simulink model "motorai"  (R2018b)
settings: Solver=FixedStepAuto  StartTime=0.0  StopTime=inf  FixedStep=SAMPLE_TIME  RelTol=1e-3
PreLoadFcn:
  | UserSettings
InitFcn:
  | ESTIMATION_SAMPLES = 50;
values from neighbouring files (symbols this model uses):
  ADC_bits = 12    [LQR_control_design.m]    (also in UserSettings.m)
  ADC_Vref = 3.3    [LQR_control_design.m]    (also in UserSettings.m)
  current_gain = 0.5    [LQR_control_design.m]    (also in UserSettings.m)
  current_offset = 1    [LQR_control_design.m]    (also in UserSettings.m)
  DATA_SAMPLING_FREQUENCY = 500    [UserSettings.m]
  K = -K    (= -0.383)    [LQG_control_design.m]    (also in LQR_control_design.m = -(1/R).*B'*Sinf; myLQR.m = -(1/R).*B'*Sinf; myREF.m = [Kw Ki])
  motorParameters = Parameters()    [UserSettings.m]
  omega_gain = 0.5    [LQR_control_design.m]    (also in UserSettings.m)
  omega_offset = 1    [LQR_control_design.m]    (also in UserSettings.m)
  PPR = 1000    [LQR_control_design.m]    (also in UserSettings.m)
  Q = 1/2*inv([(omega_max)^2 0 0; 0 (i_max)^2 0; 0 0 (int_max)^2])    [LQG_control_design.m]    (also in LQR_control_design.m = 1/2*inv([(omega_max)^2 0 ; 0 (i_max)^2]); myLQR.m = 1/2*inv([(omega_max)^2 0; 0 (i_max)^2]))
  R = inv([(v_max)^2])    [LQG_control_design.m]    (also in LQR_control_design.m; myLQR.m)
  SAMPLE_TIME = 5e-5    (= 5e-05)    [UserSettings.m]
  V_ACT = 12    [UserSettings.m]
  Vact = 12    [LQR_control_design.m]
undefined symbols (not defined in the file or in its folder): DiscIntNeverNeededParam
libraries: neural x275, mbedblockslib x7, fl_lib x5, nesl_utility x5, dspswit3 x3, elec_lib x3, powerlib_meascontrol x3, dspbuff3 x2, discretizing x1
(part 4 of 14)

== system motorai/PARAMETERS EXTIMATION HIL/Function Fitting Neural Network/Layer 2/Delays 1 ==
  "p{2}" : Inport  PortDimensions=22
      mask Display: e = 0.06;c1 = [120 230 180]/255;c2 = ([120 230 180]+0)/(256+128);c3 = ([120 230 180]+128)/(256+128);patch([0 1 1 0],[0 0 1 1],c1);patch([0 1 1 1-e 1-e 0+e],[0 0 1 1-e 0+e 0+e],c2);patch([0 0 1 1-e 0+e 0+e],[0 1 1 1-e 1-e 0+e],c3);plot([0 1 1 0 0],[0 0 1 1 0]);
  mux : Mux  Inputs=1
      mask Display: e = 0.06;c1 = [120 150 230]/255;c2 = ([120 150 230]+0)/383;c3 = ([120 150 230]+128)/383;patch([0 1 1 0],[0 0 1 1],c1);patch([0 1 1 1-e 1-e 0+e],[0 0 1 1-e 0+e 0+e],c2);patch([0 0 1 1-e 0+e 0+e],[0 1 1 1-e 1-e 0+e],c3);plot([0 1 1 0 0],[0 0 1 1 0]);disp('Mux')
  "pd{2,1}" : Outport
      mask Display: e = 0.06;c1 = [120 230 180]/255;c2 = ([120 230 180]+0)/(256+128);c3 = ([120 230 180]+128)/(256+128);patch([0 1 1 0],[0 0 1 1],c1);patch([0 1 1 1-e 1-e 0+e],[0 0 1 1-e 0+e 0+e],c2);patch([0 0 1 1-e 0+e 0+e],[0 1 1 1-e 1-e 0+e],c3);plot([0 1 1 0 0],[0 0 1 1 0]);
  wires:
  mux/1 -> "pd{2,1}"/1
  "p{2}"/1 -> mux/1

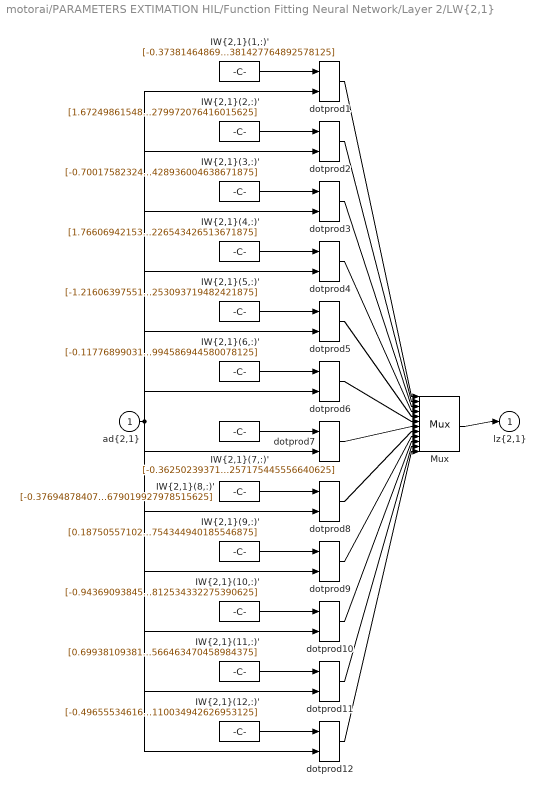
== system motorai/PARAMETERS EXTIMATION HIL/Function Fitting Neural Network/Layer 2/LW{2,1} ==
  "ad{2,1}" : Inport  PortDimensions=22
      mask Display: e = 0.06;c1 = [120 230 180]/255;c2 = ([120 230 180]+0)/(256+128);c3 = ([120 230 180]+128)/(256+128);patch([0 1 1 0],[0 0 1 1],c1);patch([0 1 1 1-e 1-e 0+e],[0 0 1 1-e 0+e 0+e],c2);patch([0 0 1 1-e 0+e 0+e],[0 1 1 1-e 1-e 0+e],c3);plot([0 1 1 0 0],[0 0 1 1 0]);
  "IW{2,1}(1,:)'" : Constant  Value=[-0.373814648698248042091307752343709580600261688232421875;2.388185086648772159634290801477618515491485595703125;0.306022187467772710522950774247874505817890167236328125;-0.74612148152227353303800327921635471284389495849609375;-0.36510707287944976773275129744433797895908355712890625;0.3483392363810693392878192753414623439311981201171875;1.0579275570388186888948212072136811912059783935546875;0.293660952316886436630483103726874105632305145263671875;2.12653508516325917554468105663545429706573486328125;0.66856009697980989248122796198003925383090972900390625;-0.51653241823746720573495849748724140226840972900390625;-0.62461964538400105428905817461782135069370269775390625;0.73347032324756289423106636604643426835536956787109375;0.60107951005838733404829099526978097856044769287109375;0.41661190433255190779249232946312986314296722412109375;-0.495062523768045215089017574427998624742031097412109375;-0.97392836170859575783964601214393042027950286865234375;-0.15328348744030317885034264691057614982128143310546875;0.955526268447108417802837720955722033977508544921875;0.30437862753427535889017008230439387261867523193359375;3.0866869361023301365776205784641206264495849609375;-0.4803399659008598110432330940966494381427764892578125]
      mask Display: e = 0.06;c1 = [120 150 230]/255;c2 = ([120 150 230]+0)/383;c3 = ([120 150 230]+128)/383;patch([0 1 1 0],[0 0 1 1],c1);patch([0 1 1 1-e 1-e 0+e],[0 0 1 1-e 0+e 0+e],c2);patch([0 0 1 1-e 0+e 0+e],[0 1 1 1-e 1-e 0+e],c3);plot([0 1 1 0 0],[0 0 1 1 0]);disp('weights');
  "IW{2,1}(10,:)'" : Constant  Value=[-0.94369093845881446558365723831229843199253082275390625;1.322843320356273721927209408022463321685791015625;0.2013525000172964596334423958978732116520404815673828125;-0.429323077932844909820886414308915846049785614013671875;0.1744635303798653114260019947323598898947238922119140625;-0.041808522872746757548245710722767398692667484283447265625;-0.210001538457013026128805677217314951121807098388671875;0.157787948169038128032326540051144547760486602783203125;-0.59934844013664434481114540176349692046642303466796875;0.0142991425154821438781027609365992248058319091796875;1.8154415812965656318311857830849476158618927001953125;-0.2181115352241077831596527403235086239874362945556640625;-0.7770603432838161239715191186405718326568603515625;0.4534919681510520828027210882282815873622894287109375;-0.237948861224295205030188071759766899049282073974609375;-1.6341662334094799735595415768329985439777374267578125;0.59471843043654015747989660667371936142444610595703125;0.727832247307649282674901769496500492095947265625;0.1267307587950488312333874318937887437641620635986328125;1.2978618628956042346800359155167825520038604736328125;-2.018836157679956944122068307478912174701690673828125;0.304437176117283991860773539883666671812534332275390625]
      mask Display: e = 0.06;c1 = [120 150 230]/255;c2 = ([120 150 230]+0)/383;c3 = ([120 150 230]+128)/383;patch([0 1 1 0],[0 0 1 1],c1);patch([0 1 1 1-e 1-e 0+e],[0 0 1 1-e 0+e 0+e],c2);patch([0 0 1 1-e 0+e 0+e],[0 1 1 1-e 1-e 0+e],c3);plot([0 1 1 0 0],[0 0 1 1 0]);disp('weights');
  "IW{2,1}(11,:)'" : Constant  Value=[0.6993810938157587475672016807948239147663116455078125;-19.28028374521506549399418872781097888946533203125;2.309346273318040321242960999370552599430084228515625;1.0652462012675394387173355426057241857051849365234375;-2.145760240313183242477634848910383880138397216796875;3.155749157418584527334814993082545697689056396484375;1.1460430072098544140857256934395991265773773193359375;-0.03602755514596193975318527691342751495540142059326171875;7.37193274662607489489118961500935256481170654296875;2.910634893704704406758310142322443425655364990234375;-2.502679544920492826776126094046048820018768310546875;5.475021714965532027008521254174411296844482421875;-2.190915873696507976120528837782330811023712158203125;0.40460150291473684358578566389041952788829803466796875;7.06424053190595113704830509959720075130462646484375;-2.498408304964217396815229221829213201999664306640625;-1.66854689838172287608131227898411452770233154296875;4.956010968949474460032433853484690189361572265625;-0.9894118095536430512737524622934870421886444091796875;3.398294550650808876213204712257720530033111572265625;-6.42259294605289188240249131922610104084014892578125;-1.01288980257130756257311077206395566463470458984375]
      mask Display: e = 0.06;c1 = [120 150 230]/255;c2 = ([120 150 230]+0)/383;c3 = ([120 150 230]+128)/383;patch([0 1 1 0],[0 0 1 1],c1);patch([0 1 1 1-e 1-e 0+e],[0 0 1 1-e 0+e 0+e],c2);patch([0 0 1 1-e 0+e 0+e],[0 1 1 1-e 1-e 0+e],c3);plot([0 1 1 0 0],[0 0 1 1 0]);disp('weights');
  "IW{2,1}(12,:)'" : Constant  Value=[-0.496555346166215938463750489972881041467189788818359375;0.00791055524906490899195166122126465779729187488555908203125;-0.11710097566626261056388358383628656156361103057861328125;-0.0165177005587808893583012803674137103371322154998779296875;-0.6454360744191973697780895236064679920673370361328125;-0.6732070109779215716372391398181207478046417236328125;0.09373162307416758876055240534697077237069606781005859375;-0.039114682492637047050987320062631624750792980194091796875;-0.1551113925473206200944531474306131713092327117919921875;-0.05012488071425476310327695728119579143822193145751953125;0.2156283243173235941725351949571631848812103271484375;-0.8022298048740685860735766254947520792484283447265625;-0.9063317432573414489382912506698630750179290771484375;-0.00032101082763222560205462752236371670733205974102020263671875;0.2671447035854070950477989754290319979190826416015625;0.69691015959264646095761008837143890559673309326171875;-0.1784561380273828878895159277817583642899990081787109375;-0.05347038743792344173133557205801480449736118316650390625;-0.11345954903014165982000349686131812632083892822265625;0.01728629936978050285478758496537921018898487091064453125;-0.85915203372011827998022681640577502548694610595703125;-1.5394571537418759721305150378611870110034942626953125]
      mask Display: e = 0.06;c1 = [120 150 230]/255;c2 = ([120 150 230]+0)/383;c3 = ([120 150 230]+128)/383;patch([0 1 1 0],[0 0 1 1],c1);patch([0 1 1 1-e 1-e 0+e],[0 0 1 1-e 0+e 0+e],c2);patch([0 0 1 1-e 0+e 0+e],[0 1 1 1-e 1-e 0+e],c3);plot([0 1 1 0 0],[0 0 1 1 0]);disp('weights');
  "IW{2,1}(2,:)'" : Constant  Value=[1.67249861548387013243655019323341548442840576171875;-0.0501570542810379771392348402514471672475337982177734375;5.45446144012502553977128627593629062175750732421875;0.3067453305420440035078399887424893677234649658203125;0.93388522037497179173470840396475978195667266845703125;0.43936786222361068343644774358836002647876739501953125;-0.72633915551496486262550433821161277592182159423828125;3.452667124378164142939340308657847344875335693359375;-1.1865375265624635847672152522136457264423370361328125;5.83346097285197284776359083480201661586761474609375;-0.7944995956295841654792866393108852207660675048828125;-1.39409214113267676538043815526179969310760498046875;-1.0713655944878925918573031594860367476940155029296875;-1.00512386920140972534909451496787369251251220703125;-1.5609895974406218233099252756801433861255645751953125;-2.43147394289584628523925857734866440296173095703125;-2.897976439331302334068141135503537952899932861328125;-2.880108124462474439297920980607159435749053955078125;11.235313175654884076948292204178869724273681640625;-1.5185828429420393792526056131464429199695587158203125;-3.28633815506999216182748568826355040073394775390625;12.7821791830810784773575505823828279972076416015625]
      mask Display: e = 0.06;c1 = [120 150 230]/255;c2 = ([120 150 230]+0)/383;c3 = ([120 150 230]+128)/383;patch([0 1 1 0],[0 0 1 1],c1);patch([0 1 1 1-e 1-e 0+e],[0 0 1 1-e 0+e 0+e],c2);patch([0 0 1 1-e 0+e 0+e],[0 1 1 1-e 1-e 0+e],c3);plot([0 1 1 0 0],[0 0 1 1 0]);disp('weights');
  "IW{2,1}(3,:)'" : Constant  Value=[-0.70017582324454863407225957416812889277935028076171875;1.67067467675322323117370615364052355289459228515625;0.1254376935351457500456007210232201032340526580810546875;-0.496595212722104661917654766511986963450908660888671875;0.094918003618071844496029143556370399892330169677734375;0.264165279391440355194475841926760040223598480224609375;-0.139597218341219797554941806083661504089832305908203125;0.117080505236092979881590281365788541734218597412109375;-0.55579337936531036934439953256514854729175567626953125;0.01236978846688709283985208031708680209703743457794189453125;1.4945214065591017060796730220317840576171875;-0.0880529371837325547378583223689929582178592681884765625;-0.7157812903296789652785037105786614120006561279296875;0.3810758435795695842074337633675895631313323974609375;-0.26285342121100196965954864936065860092639923095703125;-0.812099360289087801589857917861081659793853759765625;0.53431861847600747861264380844659171998500823974609375;0.7215442121609945136384567376808263361454010009765625;0.04721860197450167273558463421068154275417327880859375;1.1988879951099453702312302993959747254848480224609375;-3.33608458289905396298991036019288003444671630859375;-0.7836158906533199353106056150863878428936004638671875]
      mask Display: e = 0.06;c1 = [120 150 230]/255;c2 = ([120 150 230]+0)/383;c3 = ([120 150 230]+128)/383;patch([0 1 1 0],[0 0 1 1],c1);patch([0 1 1 1-e 1-e 0+e],[0 0 1 1-e 0+e 0+e],c2);patch([0 0 1 1-e 0+e 0+e],[0 1 1 1-e 1-e 0+e],c3);plot([0 1 1 0 0],[0 0 1 1 0]);disp('weights');
  "IW{2,1}(4,:)'" : Constant  Value=[1.766069421533778882604792670463211834430694580078125;1.042967917183602377662055005203001201152801513671875;-0.141883868596699047603948429241427220404148101806640625;-0.58806106441775085613699047826230525970458984375;0.311817283999389294191217913976288400590419769287109375;2.3102000569721088396590857882983982563018798828125;4.15528975409117862227503792382776737213134765625;6.21171473959054143421099070110358297824859619140625;0.1196618271109388953465924032570910640060901641845703125;0.11815122529796819039749067314915009774267673492431640625;0.9828675247137164117106067351414822041988372802734375;-1.2034037682147538106391948531381785869598388671875;-0.152664932005876163856328275869600474834442138671875;-4.595335314922895264544422389008104801177978515625;-0.6266982814945289970154362890752963721752166748046875;-1.1989185909846666877598408973426558077335357666015625;-3.6425990245676214129844083799980580806732177734375;0.123378486656041952418405571734183467924594879150390625;0.173975621097830324135458113232743926346302032470703125;-1.266562415572969779731238304520957171916961669921875;3.385659680429013551616890254081226885318756103515625;-2.130314063352613640489607860217802226543426513671875]
      mask Display: e = 0.06;c1 = [120 150 230]/255;c2 = ([120 150 230]+0)/383;c3 = ([120 150 230]+128)/383;patch([0 1 1 0],[0 0 1 1],c1);patch([0 1 1 1-e 1-e 0+e],[0 0 1 1-e 0+e 0+e],c2);patch([0 0 1 1-e 0+e 0+e],[0 1 1 1-e 1-e 0+e],c3);plot([0 1 1 0 0],[0 0 1 1 0]);disp('weights');
  "IW{2,1}(5,:)'" : Constant  Value=[-1.2160639755125342009733913073432631790637969970703125;-3.038322807923126589457751833833754062652587890625;2.95356675575607408035239132004790008068084716796875;-0.34964856620207240833764217313728295266628265380859375;-3.8401663498015086162240550038404762744903564453125;-1.434312482104028507734483355307020246982574462890625;0.498000988776814867975417655543424189090728759765625;-0.475940354291554623689108893813681788742542266845703125;0.481776521841532356926762759030680172145366668701171875;-0.0143285253932178245628303869807496084831655025482177734375;-1.62541639988879449418845979380421340465545654296875;-1.33097413271977504933829550282098352909088134765625;1.1551325139709671674381752382032573223114013671875;0.322054940956319313283273686465690843760967254638671875;0.83090978260683778788830977646284736692905426025390625;-0.9638347486264853269943841951317153871059417724609375;-0.17447941373044584256746247774572111666202545166015625;-1.6259520001337108840999690073658712208271026611328125;-0.0201962158267790063692626034708155202679336071014404296875;-2.034125459290754722729843706474639475345611572265625;7.29613836782051183860176024609245359897613525390625;-1.7639138340141122807125384497339837253093719482421875]
      mask Display: e = 0.06;c1 = [120 150 230]/255;c2 = ([120 150 230]+0)/383;c3 = ([120 150 230]+128)/383;patch([0 1 1 0],[0 0 1 1],c1);patch([0 1 1 1-e 1-e 0+e],[0 0 1 1-e 0+e 0+e],c2);patch([0 0 1 1-e 0+e 0+e],[0 1 1 1-e 1-e 0+e],c3);plot([0 1 1 0 0],[0 0 1 1 0]);disp('weights');
  "IW{2,1}(6,:)'" : Constant  Value=[-0.11776899031336483802956394129068939946591854095458984375;1.0816067725283800005087186946184374392032623291015625;-1.3725069564608916028447538337786681950092315673828125;-0.93885172581776288325272616930305957794189453125;-0.334927153732878346570345229338272474706172943115234375;3.127055083824247905255333535023964941501617431640625;3.737129929311676423964172499836422502994537353515625;6.57794136604749812846648637787438929080963134765625;0.18819194287160512235601572683663107454776763916015625;0.0062255822559748770494980618650515680201351642608642578125;1.39585907348498050595253516803495585918426513671875;-0.85890284540357908493746208478114567697048187255859375;-2.17788422026401207176604657433927059173583984375;-4.8394935373831469149763506720773875713348388671875;-0.63340718588441635716890232288278639316558837890625;-5.893111992691302702951361425220966339111328125;-2.575737579748121230949209348182193934917449951171875;0.1688019695557121391260579912341199815273284912109375;0.0131168749563965840454482503218969213776290416717529296875;-2.832832085014937550937474952661432325839996337890625;8.6321982981284204328176201670430600643157958984375;-3.655848587658077963880032257293350994586944580078125]
      mask Display: e = 0.06;c1 = [120 150 230]/255;c2 = ([120 150 230]+0)/383;c3 = ([120 150 230]+128)/383;patch([0 1 1 0],[0 0 1 1],c1);patch([0 1 1 1-e 1-e 0+e],[0 0 1 1-e 0+e 0+e],c2);patch([0 0 1 1-e 0+e 0+e],[0 1 1 1-e 1-e 0+e],c3);plot([0 1 1 0 0],[0 0 1 1 0]);disp('weights');
  "IW{2,1}(7,:)'" : Constant  Value=[-0.3625023937196261147875020469655282795429229736328125;2.741236662902159171295579653815366327762603759765625;-2.121606761392355711137724938453175127506256103515625;-0.4523900379543508432078624537098221480846405029296875;-1.433230340797343682623932181741110980510711669921875;1.878588877026521775093215183005668222904205322265625;-0.560815005670500799084265963756479322910308837890625;1.493913929936840911949502697098068892955780029296875;-3.170568963376355409167217658250592648983001708984375;4.33352532635525466986337050911970436573028564453125;-1.0881674978698507860741528929793275892734527587890625;0.5463363153126630233913374468102119863033294677734375;1.070531714404931111772611984633840620517730712890625;-0.6797290363552226377663600942469201982021331787109375;-3.36627763772676313891452082316391170024871826171875;0.131098898813111708339107508436427451670169830322265625;-1.17719923016618022160173495649360120296478271484375;3.258685294179720859375493091647513210773468017578125;5.725185804640826603417735896073281764984130859375;-1.5388387016591653644326243011164478957653045654296875;8.124922737557515262096785590983927249908447265625;3.238888438369118549786662697442807257175445556640625]
      mask Display: e = 0.06;c1 = [120 150 230]/255;c2 = ([120 150 230]+0)/383;c3 = ([120 150 230]+128)/383;patch([0 1 1 0],[0 0 1 1],c1);patch([0 1 1 1-e 1-e 0+e],[0 0 1 1-e 0+e 0+e],c2);patch([0 0 1 1-e 0+e 0+e],[0 1 1 1-e 1-e 0+e],c3);plot([0 1 1 0 0],[0 0 1 1 0]);disp('weights');
  "IW{2,1}(8,:)'" : Constant  Value=[-0.376948784072008435952483296205173246562480926513671875;-2.744608844334838426703981895116157829761505126953125;-0.354979565149837028581458753251354210078716278076171875;0.5446501025508629911797697786823846399784088134765625;0.52623456523853373578702985469135455787181854248046875;-0.4870280253021739280683277684147469699382781982421875;-0.94904641297388481202546017811982892453670501708984375;-0.27048626906591000107482614112086594104766845703125;-0.1371915607268853476430336968405754305422306060791015625;-0.5775952934599619670308356944588012993335723876953125;0.460047851461393264571597683243453502655029296875;-0.458507355789205206519909552298486232757568359375;-0.81339419741809682040667439650860615074634552001953125;-0.5181965606424674408714281526044942438602447509765625;1.446283776482689464870645679184235632419586181640625;-0.2037852020641963690650300122797489166259765625;1.03066658521672405157687535393051803112030029296875;-4.4452367691895613432961908983998000621795654296875;-0.9924712041404737394856283572153188288211822509765625;-0.19396147486783277269495329164783470332622528076171875;-2.33074689468901841138404051889665424823760986328125;2.7750555478774376894079978228546679019927978515625]
      mask Display: e = 0.06;c1 = [120 150 230]/255;c2 = ([120 150 230]+0)/383;c3 = ([120 150 230]+128)/383;patch([0 1 1 0],[0 0 1 1],c1);patch([0 1 1 1-e 1-e 0+e],[0 0 1 1-e 0+e 0+e],c2);patch([0 0 1 1-e 0+e 0+e],[0 1 1 1-e 1-e 0+e],c3);plot([0 1 1 0 0],[0 0 1 1 0]);disp('weights');
  "IW{2,1}(9,:)'" : Constant  Value=[0.1875055710261027408503053948152228258550167083740234375;0.90489674608045189696525767431012354791164398193359375;-0.12973322723757008123612877170671708881855010986328125;0.4040789428277340444850551648414693772792816162109375;0.7588494540475922978117750972160138189792633056640625;0.22043493779026090972905649323365651071071624755859375;0.091262840672618195103638072396279312670230865478515625;-0.10358510239831585086900389569564140401780605316162109375;0.48469536828752846080448080101632513105869293212890625;-0.1042448443682677805544045668284525163471698760986328125;-2.28001013511277950129851888050325214862823486328125;-0.401620072308292275220509282007697038352489471435546875;0.5889009231164286095605575610534287989139556884765625;-0.428874131242132694552537941490299999713897705078125;0.426953858134898556198066899014520458877086639404296875;3.73162300623667153587348366272635757923126220703125;-0.56022450979731319709031822640099562704563140869140625;-0.7703389604056589679004218851332552731037139892578125;-0.152647405145999337516826699356897734105587005615234375;-1.03590236727699736007934916415251791477203369140625;-0.54521841184197306073855315844411961734294891357421875;-4.37328944251520379538078486802987754344940185546875]
      mask Display: e = 0.06;c1 = [120 150 230]/255;c2 = ([120 150 230]+0)/383;c3 = ([120 150 230]+128)/383;patch([0 1 1 0],[0 0 1 1],c1);patch([0 1 1 1-e 1-e 0+e],[0 0 1 1-e 0+e 0+e],c2);patch([0 0 1 1-e 0+e 0+e],[0 1 1 1-e 1-e 0+e],c3);plot([0 1 1 0 0],[0 0 1 1 0]);disp('weights');
  Mux : Mux  Inputs=12
      mask Display: e = 0.06;c1 = [120 150 230]/255;c2 = ([120 150 230]+0)/383;c3 = ([120 150 230]+128)/383;patch([0 1 1 0],[0 0 1 1],c1);patch([0 1 1 1-e 1-e 0+e],[0 0 1 1-e 0+e 0+e],c2);patch([0 0 1 1-e 0+e 0+e],[0 1 1 1-e 1-e 0+e],c3);plot([0 1 1 0 0],[0 0 1 1 0]);disp('Mux');
  dotprod{1..12} (12 alike) : neural/Weight Functions/dotprod
      settings: SourceProductName=Deep Learning Toolbox
  "lz{2,1}" : Outport
      mask Display: e = 0.06;c1 = [120 230 180]/255;c2 = ([120 230 180]+0)/(256+128);c3 = ([120 230 180]+128)/(256+128);patch([0 1 1 0],[0 0 1 1],c1);patch([0 1 1 1-e 1-e 0+e],[0 0 1 1-e 0+e 0+e],c2);patch([0 0 1 1-e 0+e 0+e],[0 1 1 1-e 1-e 0+e],c3);plot([0 1 1 0 0],[0 0 1 1 0]);
  wires:
  Mux/1 -> "lz{2,1}"/1
  dotprod12/1 -> Mux/12
  "IW{2,1}(12,:)'"/1 -> dotprod12/1
  dotprod11/1 -> Mux/11
  "IW{2,1}(11,:)'"/1 -> dotprod11/1
  dotprod10/1 -> Mux/10
  "IW{2,1}(10,:)'"/1 -> dotprod10/1
  dotprod9/1 -> Mux/9
  "IW{2,1}(9,:)'"/1 -> dotprod9/1
  dotprod8/1 -> Mux/8
  "IW{2,1}(8,:)'"/1 -> dotprod8/1
  dotprod7/1 -> Mux/7
  "IW{2,1}(7,:)'"/1 -> dotprod7/1
  dotprod6/1 -> Mux/6
  "IW{2,1}(6,:)'"/1 -> dotprod6/1
  dotprod5/1 -> Mux/5
  "IW{2,1}(5,:)'"/1 -> dotprod5/1
  dotprod4/1 -> Mux/4
  "IW{2,1}(4,:)'"/1 -> dotprod4/1
  dotprod3/1 -> Mux/3
  "IW{2,1}(3,:)'"/1 -> dotprod3/1
  dotprod2/1 -> Mux/2
  "IW{2,1}(2,:)'"/1 -> dotprod2/1
  dotprod1/1 -> Mux/1
  "ad{2,1}"/1 -> dotprod12/2, dotprod11/2, dotprod10/2, dotprod9/2, dotprod8/2, dotprod7/2, dotprod6/2, dotprod5/2, dotprod4/2, dotprod3/2, dotprod2/2, dotprod1/2
  "IW{2,1}(1,:)'"/1 -> dotprod1/1

== system motorai/PARAMETERS EXTIMATION HIL/Function Fitting Neural Network/Layer 3/Delays 1 ==
  "p{3}" : Inport  PortDimensions=12
      mask Display: e = 0.06;c1 = [120 230 180]/255;c2 = ([120 230 180]+0)/(256+128);c3 = ([120 230 180]+128)/(256+128);patch([0 1 1 0],[0 0 1 1],c1);patch([0 1 1 1-e 1-e 0+e],[0 0 1 1-e 0+e 0+e],c2);patch([0 0 1 1-e 0+e 0+e],[0 1 1 1-e 1-e 0+e],c3);plot([0 1 1 0 0],[0 0 1 1 0]);
  mux : Mux  Inputs=1
      mask Display: e = 0.06;c1 = [120 150 230]/255;c2 = ([120 150 230]+0)/383;c3 = ([120 150 230]+128)/383;patch([0 1 1 0],[0 0 1 1],c1);patch([0 1 1 1-e 1-e 0+e],[0 0 1 1-e 0+e 0+e],c2);patch([0 0 1 1-e 0+e 0+e],[0 1 1 1-e 1-e 0+e],c3);plot([0 1 1 0 0],[0 0 1 1 0]);disp('Mux')
  "pd{3,2}" : Outport
      mask Display: e = 0.06;c1 = [120 230 180]/255;c2 = ([120 230 180]+0)/(256+128);c3 = ([120 230 180]+128)/(256+128);patch([0 1 1 0],[0 0 1 1],c1);patch([0 1 1 1-e 1-e 0+e],[0 0 1 1-e 0+e 0+e],c2);patch([0 0 1 1-e 0+e 0+e],[0 1 1 1-e 1-e 0+e],c3);plot([0 1 1 0 0],[0 0 1 1 0]);
  wires:
  mux/1 -> "pd{3,2}"/1
  "p{3}"/1 -> mux/1

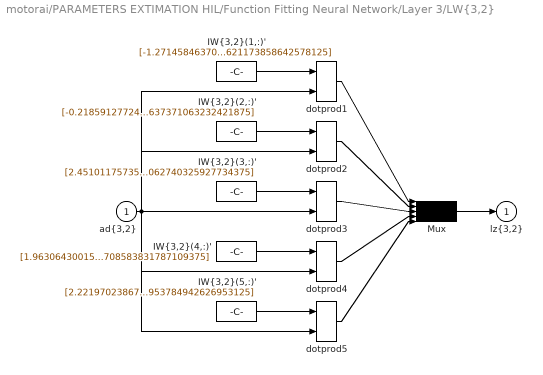
== system motorai/PARAMETERS EXTIMATION HIL/Function Fitting Neural Network/Layer 3/LW{3,2} ==
  "ad{3,2}" : Inport  PortDimensions=12
      mask Display: e = 0.06;c1 = [120 230 180]/255;c2 = ([120 230 180]+0)/(256+128);c3 = ([120 230 180]+128)/(256+128);patch([0 1 1 0],[0 0 1 1],c1);patch([0 1 1 1-e 1-e 0+e],[0 0 1 1-e 0+e 0+e],c2);patch([0 0 1 1-e 0+e 0+e],[0 1 1 1-e 1-e 0+e],c3);plot([0 1 1 0 0],[0 0 1 1 0]);
  "IW{3,2}(1,:)'" : Constant  Value=[-1.271458463700293695097798263304866850376129150390625;-0.8974504950343582532212849400821141898632049560546875;-1.7160155942908417170400525719742290675640106201171875;3.778124449975665211098885265528224408626556396484375;1.0463511136165484227689148610807023942470550537109375;-4.198289194390252276889441418461501598358154296875;2.185971342736543032714280343498103320598602294921875;-1.562305785175263306285842190845869481563568115234375;2.086082505458115132768170951749198138713836669921875;3.74283631710132880243691033683717250823974609375;0.50886956911632552635893489423324353992938995361328125;2.005558951607021800356278617982752621173858642578125]
      mask Display: e = 0.06;c1 = [120 150 230]/255;c2 = ([120 150 230]+0)/383;c3 = ([120 150 230]+128)/383;patch([0 1 1 0],[0 0 1 1],c1);patch([0 1 1 1-e 1-e 0+e],[0 0 1 1-e 0+e 0+e],c2);patch([0 0 1 1-e 0+e 0+e],[0 1 1 1-e 1-e 0+e],c3);plot([0 1 1 0 0],[0 0 1 1 0]);disp('weights');
  "IW{3,2}(2,:)'" : Constant  Value=[-0.2185912772434949469246845410452806390821933746337890625;2.780442287080636898366492459899745881557464599609375;-7.1433250739280982344325821031816303730010986328125;-5.8302706988147026123670002561993896961212158203125;-1.2314158784646254130024090045480988919734954833984375;7.163539222352397928261780180037021636962890625;-3.523963080517721113693596635130234062671661376953125;-0.061199348948568786654700346616664319299161434173583984375;-2.882119860196695082521500808070413768291473388671875;3.8358372116914747351756886928342282772064208984375;0.50841029127393955189262442218023352324962615966796875;1.5784512378830235501681045207078568637371063232421875]
      mask Display: e = 0.06;c1 = [120 150 230]/255;c2 = ([120 150 230]+0)/383;c3 = ([120 150 230]+128)/383;patch([0 1 1 0],[0 0 1 1],c1);patch([0 1 1 1-e 1-e 0+e],[0 0 1 1-e 0+e 0+e],c2);patch([0 0 1 1-e 0+e 0+e],[0 1 1 1-e 1-e 0+e],c3);plot([0 1 1 0 0],[0 0 1 1 0]);disp('weights');
  "IW{3,2}(3,:)'" : Constant  Value=[2.451011757354031761479973283712752163410186767578125;1.6157664943008518410039187074289657175540924072265625;-0.61929996676544696310173776510055176913738250732421875;-2.62854204907607336139108156203292310237884521484375;2.108035044305257343921766732819378376007080078125;1.16718044073292848139544730656780302524566650390625;-2.93462821866088052757959303562529385089874267578125;2.684585344176590115949920800630934536457061767578125;0.6897364749097223413087931476184166967868804931640625;1.2923000217448075144233143873861990869045257568359375;-0.48945753844226180806487036534235812723636627197265625;-2.854344740097070509676768779172562062740325927734375]
      mask Display: e = 0.06;c1 = [120 150 230]/255;c2 = ([120 150 230]+0)/383;c3 = ([120 150 230]+128)/383;patch([0 1 1 0],[0 0 1 1],c1);patch([0 1 1 1-e 1-e 0+e],[0 0 1 1-e 0+e 0+e],c2);patch([0 0 1 1-e 0+e 0+e],[0 1 1 1-e 1-e 0+e],c3);plot([0 1 1 0 0],[0 0 1 1 0]);disp('weights');
  "IW{3,2}(4,:)'" : Constant  Value=[1.9630643001561711713520708144642412662506103515625;5.84020585516511392398797397618182003498077392578125;0.803446280706621163147929109982214868068695068359375;-2.073434273153257567656737592187710106372833251953125;5.49585658359518447468872182071208953857421875;0.9007634491038600810242087391088716685771942138671875;-0.52604666702190427951535411921213380992412567138671875;2.180923917199018458035197909339331090450286865234375;-0.39194927482752450753622497359174303710460662841796875;-1.2812498988512281972163009413634426891803741455078125;7.45228919574556680771593164536170661449432373046875;-6.04501097450363200636047622538171708583831787109375]
      mask Display: e = 0.06;c1 = [120 150 230]/255;c2 = ([120 150 230]+0)/383;c3 = ([120 150 230]+128)/383;patch([0 1 1 0],[0 0 1 1],c1);patch([0 1 1 1-e 1-e 0+e],[0 0 1 1-e 0+e 0+e],c2);patch([0 0 1 1-e 0+e 0+e],[0 1 1 1-e 1-e 0+e],c3);plot([0 1 1 0 0],[0 0 1 1 0]);disp('weights');
  "IW{3,2}(5,:)'" : Constant  Value=[2.2219702386759383472281115246005356311798095703125;-9.289596730222655196484993211925029754638671875;0.6645354413043247365777688173693604767322540283203125;-6.64663738028603834351315526873804628849029541015625;-3.38309296602343945181701201363466680049896240234375;5.69637196720368166324988123960793018341064453125;4.39668054474418656951684170053340494632720947265625;2.532867075917488275393907315446995198726654052734375;1.1072490285534366538655604017549194395542144775390625;-0.5005871972185220730722221560426987707614898681640625;-0.292612600291744850977693204185925424098968505859375;-4.174617596875805247691459953784942626953125]
      mask Display: e = 0.06;c1 = [120 150 230]/255;c2 = ([120 150 230]+0)/383;c3 = ([120 150 230]+128)/383;patch([0 1 1 0],[0 0 1 1],c1);patch([0 1 1 1-e 1-e 0+e],[0 0 1 1-e 0+e 0+e],c2);patch([0 0 1 1-e 0+e 0+e],[0 1 1 1-e 1-e 0+e],c3);plot([0 1 1 0 0],[0 0 1 1 0]);disp('weights');
  Mux : Mux  Inputs=5
      mask Display: e = 0.06;c1 = [120 150 230]/255;c2 = ([120 150 230]+0)/383;c3 = ([120 150 230]+128)/383;patch([0 1 1 0],[0 0 1 1],c1);patch([0 1 1 1-e 1-e 0+e],[0 0 1 1-e 0+e 0+e],c2);patch([0 0 1 1-e 0+e 0+e],[0 1 1 1-e 1-e 0+e],c3);plot([0 1 1 0 0],[0 0 1 1 0]);disp('Mux');
  dotprod{1..5} (5 alike) : neural/Weight Functions/dotprod
      settings: SourceProductName=Deep Learning Toolbox
  "lz{3,2}" : Outport
      mask Display: e = 0.06;c1 = [120 230 180]/255;c2 = ([120 230 180]+0)/(256+128);c3 = ([120 230 180]+128)/(256+128);patch([0 1 1 0],[0 0 1 1],c1);patch([0 1 1 1-e 1-e 0+e],[0 0 1 1-e 0+e 0+e],c2);patch([0 0 1 1-e 0+e 0+e],[0 1 1 1-e 1-e 0+e],c3);plot([0 1 1 0 0],[0 0 1 1 0]);
  wires:
  Mux/1 -> "lz{3,2}"/1
  dotprod5/1 -> Mux/5
  "IW{3,2}(5,:)'"/1 -> dotprod5/1
  dotprod4/1 -> Mux/4
  "IW{3,2}(4,:)'"/1 -> dotprod4/1
  dotprod3/1 -> Mux/3
  "IW{3,2}(3,:)'"/1 -> dotprod3/1
  dotprod2/1 -> Mux/2
  "IW{3,2}(2,:)'"/1 -> dotprod2/1
  dotprod1/1 -> Mux/1
  "ad{3,2}"/1 -> dotprod5/2, dotprod4/2, dotprod3/2, dotprod2/2, dotprod1/2
  "IW{3,2}(1,:)'"/1 -> dotprod1/1

== system motorai/Parameter Estimation & LQR /Function Fitting Neural Network1/Layer 1/Delays 1 ==
  "p{1}" : Inport  PortDimensions=100
      mask Display: e = 0.06;c1 = [120 230 180]/255;c2 = ([120 230 180]+0)/(256+128);c3 = ([120 230 180]+128)/(256+128);patch([0 1 1 0],[0 0 1 1],c1);patch([0 1 1 1-e 1-e 0+e],[0 0 1 1-e 0+e 0+e],c2);patch([0 0 1 1-e 0+e 0+e],[0 1 1 1-e 1-e 0+e],c3);plot([0 1 1 0 0],[0 0 1 1 0]);
  mux : Mux  Inputs=1
      mask Display: e = 0.06;c1 = [120 150 230]/255;c2 = ([120 150 230]+0)/383;c3 = ([120 150 230]+128)/383;patch([0 1 1 0],[0 0 1 1],c1);patch([0 1 1 1-e 1-e 0+e],[0 0 1 1-e 0+e 0+e],c2);patch([0 0 1 1-e 0+e 0+e],[0 1 1 1-e 1-e 0+e],c3);plot([0 1 1 0 0],[0 0 1 1 0]);disp('Mux')
  "pd{1,1}" : Outport
      mask Display: e = 0.06;c1 = [120 230 180]/255;c2 = ([120 230 180]+0)/(256+128);c3 = ([120 230 180]+128)/(256+128);patch([0 1 1 0],[0 0 1 1],c1);patch([0 1 1 1-e 1-e 0+e],[0 0 1 1-e 0+e 0+e],c2);patch([0 0 1 1-e 0+e 0+e],[0 1 1 1-e 1-e 0+e],c3);plot([0 1 1 0 0],[0 0 1 1 0]);
  wires:
  "p{1}"/1 -> mux/1
  mux/1 -> "pd{1,1}"/1
